simulink library "SimWindFarm_lib"  (Simulink 10.3)
settings: Solver=ode45  StartTime=0.0  StopTime=10.0  RelTol=1e-3  EnableMultiTasking=on
undefined symbols (not defined in the file): sigbuilder_block
libraries: simulink x3
(part 1 of 2)
settings Model: Creator=grunnet  LastModifiedBy=yerai
settings Model: SuppressorTable=|
  | <?xml version="1.0" encoding="UTF-8" standalone="yes" ?>
  | <!DOCTYPE boost_serialization>
  | <boost_serialization signature="serialization::archive" version="17">
  | <DiagnosticSuppressor class_id="0" tracking_level="0" version="7">
  | 	<Table class_id="1" tracking_level="0" version="0">
  | 		<count>3</count>
  | 		<bucket_count>8</bucket_count>
  | 		<item_version>0</item_version>
  | 		<item class_id="2" tracking_level="0" version="0">
  | 			<first class_id="3" tracking_level="0" version="7">
  | 				<Source class_id="4" tracking_level="0" version="0">
  | 					<count>1</count>
  | 					<item_version>0</item_version>
  | 					<item>183</item>
  | 				</Source>
  | 			</first>
  | 			<second class_id="5" tracking_level="0" version="7">
  | 				<SuppressedData class_id="6" tracking_level="0" version="0">
  | 					<count>2</count>
  | 					<bucket_count>8</bucket_count>
  | 					<item_version>0</item_version>
  | 					<item class_id="7" tracking_level="0" version="0">
  | 						<first class_id="8" tracking_level="0" version="7">
  | 							<ID>SimulinkFixedPoint:util:Overflowoccurred</ID>
  | 							<Cause>
  | 								<Source>
  | 									<count>0</count>
  | 									<item_version>0</item_version>
  | 								</Source>
  | 							</Cause>
  | 						</first>
  | 						<second class_id="9" tracking_level="0" version="7">
  | 							<Comment></Comment>
  | 							<User></User>
  | 							<LastModified class_id="10" tracking_level="0" version="0">
  | 								<ptime_date class_id="11" tracking_level="0" version="0">
  | 									<date>20160523</date>
  | 								</ptime_date>
  | 								<ptime_time_duration class_id="12" tracking_level="0" version="1">
  | 									<is_special>0</is_special>
  | 									<time_duration_hours>10</time_duration_hours>
  | 									<time_duration_minutes>57</time_duration_minutes>
  | 									<time_duration_seconds>55</time_duration_seconds>
  | 									<time_duration_fractional_seconds>0</time_duration_fractional_seconds>
  | 								</ptime_time_duration>
  | 							</LastModified>
  | 							<SuppressionType>1</SuppressionType>
  | 						</second>
  | 					</item>
  | 					<item>
  | 						<first>
  | 							<ID>Simulink:DataType:WarningOverFlowDetected</ID>
  | 							<Cause>
  | 								<Source>
  | 									<count>0</count>
  | 									<item_version>0</item_version>
  | 								</Source>
  | 							</Cause>
  | 						</first>
  | 						<second>
  | 							<Comment></Comment>
  | 							<User></User>
  | 							<LastModified>
  | 								<ptime_date>
  | 									<date>20160523</date>
  | 								</ptime_date>
  | 								<ptime_time_duration>
  | 									<is_special>0</is_special>
  | 									<time_duration_hours>10</time_duration_hours>
  | 									<time_duration_minutes>57</time_duration_minutes>
  | 									<time_duration_seconds>55</time_duration_seconds>
  | 									<time_duration_fractional_seconds>0</time_duration_fractional_seconds>
  | 								</ptime_time_duration>
  | 							</LastModified>
  | 							<SuppressionType>1</SuppressionType>
  | 						</second>
  | 					</item>
  | 				</SuppressedData>
  | 			</second>
  | 		</item>
  | 		<item>
  | 			<first>
  | 				<Source>
  | 					<count>1</count>
  | 					<item_version>0</item_version>
  | 					<item>243:183</item>
  | 				</Source>
  | 			</first>
  | 			<second>
  | 				<SuppressedData>
  | 					<count>2</count>
  | 					<bucket_count>8</bucket_count>
  | 					<item_version>0</item_version>
  | 					<item>
  | 						<first>
  | 							<ID>SimulinkFixedPoint:util:Overflowoccurred</ID>
  | 							<Cause>
  | 								<Source>
  | 									<count>0</count>
  | 									<item_version>0</item_version>
  | 								</Source>
  | 							</Cause>
  | 						</first>
  | 						<second>
  | 							<Comment></Comment>
  | 							<User></User>
  | 							<LastModified>
  | 								<ptime_date>
  | 									<date>20160523</date>
  | 								</ptime_date>
  | 								<ptime_time_duration>
  | 									<is_special>0</is_special>
  | 									<time_duration_hours>10</time_duration_hours>
  | 									<time_duration_minutes>57</time_duration_minutes>
  | 									<time_duration_seconds>55</time_duration_seconds>
  | 									<time_duration_fractional_seconds>0</time_duration_fractional_seconds>
  | 								</ptime_time_duration>
  | 							</LastModified>
  | 							<SuppressionType>1</SuppressionType>
  | 						</second>
  | 					</item>
  | 					<item>
  | 						<first>
  | 							<ID>Simulink:DataType:WarningOverFlowDetected</ID>
  | 							<Cause>
  | 								<Source>
  | 									<count>0</count>
  | 									<item_version>0</item_version>
  | 								</Source>
  | 							</Cause>
  | 						</first>
  | 						<second>
  | 							<Comment></Comment>
  | 							<User></User>
  | 							<LastModified>
  | 								<ptime_date>
  | 									<date>20160523</date>
  | 								</ptime_date>
  | 								<ptime_time_duration>
  | 									<is_special>0</is_special>
  | 									<time_duration_hours>10</time_duration_hours>
  | 									<time_duration_minutes>57</time_duration_minutes>
  | 									<time_duration_seconds>55</time_duration_seconds>
  | 									<time_duration_fractional_seconds>0</time_duration_fractional_seconds>
  | 								</ptime_time_duration>
  | 							</LastModified>
  | 							<SuppressionType>1</SuppressionType>
  | 						</second>
  | 					</item>
  | 				</SuppressedData>
  | 			</second>
  | 		</item>
  | 		<item>
  | 			<first>
  | 				<Source>
  | 					<count>1</count>
  | 					<item_version>0</item_version>
  | 					<item>80</item>
  | 				</Source>
  | 			</first>
  | 			<second>
  | 				<SuppressedData>
  | 					<count>2</count>
  | 					<bucket_count>8</bucket_count>
  | 					<item_version>0</item_version>
  | 					<item>
  | 						<first>
  | 							<ID>SimulinkFixedPoint:util:Overflowoccurred</ID>
  | 							<Cause>
  | 								<Source>
  | 									<count>0</count>
  | 									<item_version>0</item_version>
  | 								</Source>
  | 							</Cause>
  | 						</first>
  | 						<second>
  | 							<Comment></Comment>
  | 							<User></User>
  | 							<LastModified>
  | 								<ptime_date>
  | 									<date>20160523</date>
  | 								</ptime_date>
  | 								<ptime_time_duration>
  | 									<is_special>0</is_special>
  | 									<time_duration_hours>10</time_duration_hours>
  | 									<time_duration_minutes>57</time_duration_minutes>
  | 									<time_duration_seconds>55</time_duration_seconds>
  | 									<time_duration_fractional_seconds>0</time_duration_fractional_seconds>
  | 								</ptime_time_duration>
  | 							</LastModified>
  | 							<SuppressionType>1</SuppressionType>
  | 						</second>
  | 					</item>
  | 					<item>
  | 						<first>
  | 							<ID>Simulink:DataType:WarningOverFlowDetected</ID>
  | 							<Cause>
  | 								<Source>
  | 									<count>0</count>
  | 									<item_version>0</item_version>
  | 								</Source>
  | 							</Cause>
  | 						</first>
  | 						<second>
  | 							<Comment></Comment>
  | 							<User></User>
  | 							<LastModified>
  | 								<ptime_date>
  | 									<date>20160523</date>
  | 								</ptime_date>
  | 								<ptime_time_duration>
  | 									<is_special>0</is_special>
  | 									<time_duration_hours>10</time_duration_hours>
  | 									<time_duration_minutes>57</time_duration_minutes>
  | 									<time_duration_seconds>55</time_duration_seconds>
  | 									<time_duration_fractional_seconds>0</time_duration_fractional_seconds>
  | 								</ptime_time_duration>
  | 							</LastModified>
  | 							<SuppressionType>1</SuppressionType>
  | 						</second>
  | 					</item>
  | 				</SuppressedData>
  | 			</second>
  | 		</item>
  | 	</Table>
  | </DiagnosticSuppressor>
  | 
  | </boost_serialization>
  | 
  | </boost_serialization>

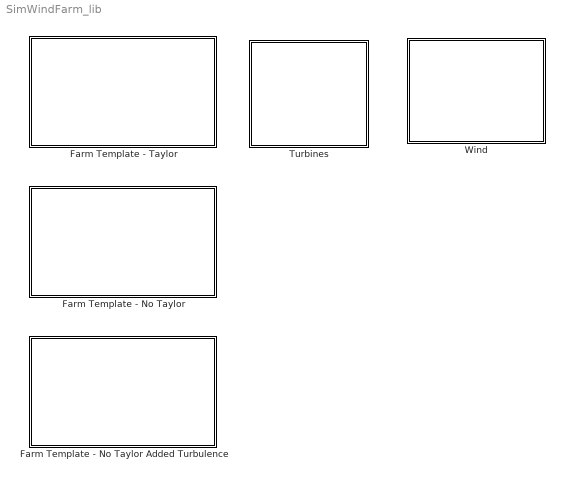
== system SimWindFarm_lib ==
  Farm Template - No Taylor : Subsystem  mask(Aeolus){}
      mask help: Wind Farm Template for the Aeolus Farm Simulator.
      settings: OpenFcn=create_windfarm_no_taylor()
      mask Display: image(imread('farm.jpg'))
  Farm Template - No Taylor Added Turbulence : Subsystem  AncestorBlock=libaeolus_at/Farm Template - No Taylor  mask(Aeolus){}
      mask help: Wind Farm Template for the Aeolus Farm Simulator.
      settings: OpenFcn=create_windfarm_no_taylor()
      mask Display: image(imread('farm.jpg'))
  Farm Template - Taylor : Subsystem  mask(Aeolus){}
      mask help: Wind Farm Template for the Aeolus Farm Simulator.
      settings: OpenFcn=create_windfarm()
      mask Display: image(imread('farm.jpg'))
  Turbines : Subsystem
      settings: OpenFcn=libturbines
      mask Display: image(imread('tblib.jpg'))
  Wind : Subsystem
      settings: OpenFcn=libwind
      mask Display: image(imread('wind.jpg'))

== system SimWindFarm_lib/Farm Template - No Taylor ==
  Farm Control : Subsystem  mask(Farm Control){Ts=5}
      mask prompts: Ts "Control Sample Time"
      mask help: A Farm controller with proportional distribution
      mask init:
      | parm=get_param(gcb,'UserData');
      | CTs=Ts;
      mask Display:
      | color('black')
      | port_label('input',1,'P_meas [W]')
      | port_label('input',2,'V_meas [m/s]')
      | port_label('input',3,'w_rot [rad/s]')
      | port_label('input',4,'Pitch [deg]')
      | port_label('input',5,'Aux')
      | port_label('input',6,'P_farm_dem [W]')
      | 
      | 
      | port_label('output',1,'P_dem[W]')
      | port_label('output',2,'P_avail [W]')
  Grid : Subsystem  mask{fgain=2e-9}
      mask prompts: fgain "Power to frequency gain"
      mask init:
      | frequencygain=fgain;
      mask Display:
      | image(imread('grid.jpg'))
      | 
      | port_label('input',1,'P_farm [W]')
      | port_label('input',2,'P_grid [W]')
      | port_label('output',1,'f_grid [Hz]')
  Network Load : Subsystem  mask{maxp=15e6}
      mask prompts: maxp "Max farm power [W]"
      mask init:
      | maxpower=maxp;
      mask Display:
      | image(imread('load.png'))
      | 
      | port_label('output',1,'P_grid[W]')
  Network Operator : Subsystem  mask{mode=Absolute, Ts=30, pref=12e6, rate=1e6, delta=2e6, db=.1, cb=1, maxp=15e6, minp=10e6, freq=50, delay=.1}
      mask prompts: mode "Operating Mode"; Ts "Sample Time [s]"; pref "Power reference [W]"; rate "Power rate limit [W/s]"; delta "Reserved power [W]"; db "Dead band [Hz]"; cb "Control band [Hz]"; maxp "Maximum power [W]"; minp "Minimum power [W]"; freq "Frequency reference [Hz]"; delay "Communication delay [s]"
      mask help: Network Operator Parameters
      mask init:
      | parm.Ts=Ts;
      | parm.mode=mode;
      | switch(mode)
      |     case 1
      |         parm.settings(1)=pref;
      |     case 2
      |         parm.settings(1)=delta;
      |     case 3
      |         parm.settings(1)=pref;
      |     case 4
      |         parm.settings(1)=rate;
      |     case 5
      |         parm.settings(1)=db;
      |         parm.settings(2)=cb;
      |         parm.settings(3)=maxp;
      |         parm.settings(4)=minp;
      |         parm.settings(5)=freq;
      |     otherwise
      |         parm.settings(1)=1e10;
      | end
      | parm.delay=delay;
      mask TypeOptions mode: Absolute | Delta | Balance | Rate Limit | Frequency
      mask Callback mode:
      | m=get_param(gcb,'mode');
      | switch(m)
      |     case 'Absolute'
      |         mv={'on','on','on','off','off', ...
      |             'off','off','off','off','off','on'};
      |     case 'Delta'
      |         mv={'on','on','off','off','on', ...
      |             'off','off','off','off','off','on'};
      |     case 'Balance'
      |         mv={'on','on','on','off','off', ...
      |             'off','off','off','off','off','on'};
      |     case 'Rate Limit'
      |         mv={'on','on','off','on','off', ...
      |             'off','off','off','off','off','on'};
      |     case 'Frequency'
      |         mv={'on','on','off','off','off', ...
      |             'on','on','on','on','on','on'};
      | end
      | 
      | set_param(gcb,'MaskVisibilities',mv);
      mask Display:
      | port_label('output',1,'P_farm_dem [W]')
      | port_label('input',1,'P_avail[W]')
      | port_label('input',2,'f_grid [Hz]')
  Post processing : Subsystem
      mask Display: image(imread('postproc.png'))
  Total power : Sum  Inputs=+
  Turbines : Subsystem  LoadFcn=|  mask(Data logging setup){mode=Wind Sync, ts=-1, dec=1}
      | p=get_param(gcb,'UserData');                                                                                                                                            
      | %If not compatible                                                                                                                                                      
      |                                                                                                                                                                         
      | %Check to avoid template warning                                                                                                                                        
      | if(~isempty(p))                                                                                                                                                         
      |                                                                                                                                                                         
      | 	if(~iscompat(p.version))                                                                                                                                               
      | 		warndlg('The version of SimWindFarm used to create this model does not match the installed version! This may result in undefined behaviour.','Model version mismatch')
      | 	end                                                                                                                                                                    
      | end
      mask prompts: mode "Sample Mode"; ts "Sample Time"; dec "Decimation"
      mask help: Adjust the amount of data logged from the turbines
      mask init:
      | switch(mode)
      |     case 3 %inherit
      |         TTs=-1;
      |     case 1 %Wind
      |         TTs=str2num(get_param([bdroot '/Wind Field/CTrate'],'OutPortSampleTime'));
      |     case 2 %costum
      |         TTs=ts;
      | end
      | 
      | assignin('base','SWFdecimation',dec);
      | assignin('base','SWFTTs',TTs);
      mask Help:
      | Wind Synch - Data is logged with the wind field time step
      | Specify - Set a custom sampling time
      | Inherit - Inherit from output port
      mask TypeOptions mode: Wind Sync | Specify | Inherit
      mask Callback mode:
      | m=get_param(gcb,'mode');
      | switch(m)
      |     case 'Specify'
      |         mv={'on','on','on'};
      |     otherwise %case 'Wind Sync'
      |         mv={'on','off','on'};
      | end
      | 
      | set_param(gcb,'MaskVisibilities',mv);
      mask Display:
      | image(imread('tblib.jpg'))
      | port_label('input',1,'P_dem [W]')
      | port_label('input',2,'V_rot [m/s]')
      | port_label('input',3,'V_nac [m/s]')
      | port_label('output',1,'P [W]')
      | port_label('output',2,'V_meas [m/s]')
      | port_label('output',3,'w_gen [m/s]')
      | port_label('output',4,'Pitch [deg]')
      | port_label('output',5,'Aux')
      | port_label('output',6,'CT')
  Wind Field : Subsystem
      mask init:
      | p=get_param(gcb,'UserData');
      settings: OpenFcn=|
      | [wfile,wpath,wfidx]=uigetfile('*.mat','Select a Wind Data File');
      | if isequal(wfile,0) || isequal(wpath,0)
      |    return
      | end
      | 
      | %Loads wind profile data
      | l=load([wpath wfile]);
      | p=get_param([gcb '/Ambient Lateral Field'],'UserData');
      | 
      | %Check for compatible wind field
      | if (~isequal(p.grid,l.wind.grid))
      |     str_grids = sprintf('\n            Model     New wind \n size          %d         %d \n xsize       %d       %d \n ysize        %d      %d \n \n Try to type: help create_windfield_no_taylor',p.grid.size, l.wind.grid.size, p.grid.xsize, l.wind.grid.xsize, p.grid.ysize, l.wind.grid.ysize);
      |     errordlg(['The wind fields must have the same grid' str_grids],'Wind field Error')
      |    return
      | end
      | 
      | %Check for correct wind field type
      | if(~isfield(l.wind,'ambient_wind'))
      |     errordlg('It is not the correct wind field type. Probably a normal taylor wind field. See create_windfield_no_taylor()','Wind field invalid')
      |    return
      | end
      | 
      | %Check compatible mean wind speed
      | if(~isfield(l.wind,'Umean') | ~isfield(p,'Umean'))
      |     warning('WarnTests:convertTest','Mean wind speed is not part of wind field struct.\n Consider updating model or windfield to newest version of SimWindFarm \n To get correct simulation behaviour, the mean wind speed of the wind field needs to be equal to the one used when farm model is created')
      | else
      |     if (~isequal(p.Umean,l.wind.Umean))
      |         str_wind_speeds = sprintf('Old mean wind speed (%d m/s) does not correspond to new mean wind speed (%d m/s). \n This may cause the simulation to be incorrect because wake delay between turbines changes. \n The solution is to create a new model with the desired average wind speed. \n Setting new windfield anyway.....', p.Umean, l.wind.Umean);
      |         warndlg(str_wind_speeds, 'Mean wind speed incompatibility')
      |     end
      | end
      | 
      | 
      | 
      | if(~isequal(p.ambient_wind.wind_pos,l.wind.ambient_wind.wind_pos))
      |   errordlg('The turbines must have same position','Wind field Error')
      |    return
      | end
      | 
      | %If the wind field is too short, reset the simulation time
      | if(p.SimTime < eval(get_param(bdroot,'StopTime')))
      |     warndlg('The model simulation time is longer than windfield. Resetting model simulation time')
      |     set_param(bdroot,'StopTime',num2str(p.SimTime))
      | end
      | 
      | 
      | %Change wf sample time
      | set_param([gcb '/CTrate'],'OutPortSampleTime',num2str(l.wind.Ts))
      | 
      | %Add old turbine position data
      | l.wind.xgrids=p.xgrids;
      | 
      | %Save the new parameters
      | set_param([gcb '/Ambient Lateral Field'],'UserData',l.wind);
      | for i=1:length(p.ambient_wind.turb_pos)
      |   pp = get_param([gcb '/Wind Speed'   num2str(i)],'UserData');
      |   pp_new = pp;
      |   pp_new.wind = l.wind.ambient_wind.wind{i};
      |   set_param([gcb '/Wind Speed' num2str(i)],'UserData',pp_new);
      | end
      mask Display:
      | image(imread('wind.jpg'))
      | 
      | port_label('input',1,'CT')
      | port_label('output',1,'V_nac [m/s]')
      | port_label('output',2,'V_rot [m/s]')
  wires:
  Turbines/3(w_gen) -> Farm Control/3(w_rot [rad/s])
  Turbines/4(pitch) -> Farm Control/4(Pitch [deg])
  Turbines/5(aux) -> Farm Control/5(" Aux")
  Network Load/1(Power Consumption [W]) -> Grid/2(Consumed Power [W])
  Total power/1 -> Grid/1(Generated Power [W])
  Grid/1(Grid Frequency [Hz]) -> Network Operator/2(Freq [Hz])
  Network Operator/1(P_farm [W]) -> Farm Control/6(P_farm [W])
  Farm Control/2(P_avail [W]) -> Network Operator/1(P_avail [W])
  Turbines/1(P) -> Farm Control/1(P_meas [W]), Total power/1
  Turbines/2(V_nac_meas [m/s]) -> Farm Control/2(V_meas [m/s])
  Farm Control/1(P_dem [W]) -> Turbines/1(P_dem [W])
  Wind Field/2(V_rot) -> Turbines/2(V_rot [m/s])
  Wind Field/1(V_nac) -> Turbines/3(V_nac [m/s])
  Turbines/6(CT) -> Wind Field/1(CT)

== system SimWindFarm_lib/Farm Template - No Taylor Added Turbulence ==
  Farm Control : Subsystem  mask(Farm Control){Ts=5}
      mask prompts: Ts "Control Sample Time"
      mask help: A Farm controller with proportional distribution
      mask init:
      | parm=get_param(gcb,'UserData');
      | CTs=Ts;
      mask Display:
      | color('black')
      | port_label('input',1,'P_meas [W]')
      | port_label('input',2,'V_meas [m/s]')
      | port_label('input',3,'w_rot [rad/s]')
      | port_label('input',4,'Pitch [deg]')
      | port_label('input',5,'Aux')
      | port_label('input',6,'P_farm_dem [W]')
      | 
      | 
      | port_label('output',1,'P_dem[W]')
      | port_label('output',2,'P_avail [W]')
  Grid : Subsystem  mask{fgain=2e-9}
      mask prompts: fgain "Power to frequency gain"
      mask init:
      | frequencygain=fgain;
      mask Display:
      | image(imread('grid.jpg'))
      | 
      | port_label('input',1,'P_farm [W]')
      | port_label('input',2,'P_grid [W]')
      | port_label('output',1,'f_grid [Hz]')
  Network Load : Subsystem  mask{maxp=15e6}
      mask prompts: maxp "Max farm power [W]"
      mask init:
      | maxpower=maxp;
      mask Display:
      | image(imread('load.png'))
      | 
      | port_label('output',1,'P_grid[W]')
  Network Operator : Subsystem  mask{mode=Absolute, Ts=30, pref=12e6, rate=1e6, delta=2e6, db=.1, cb=1, maxp=15e6, minp=10e6, freq=50, delay=.1}
      mask prompts: mode "Operating Mode"; Ts "Sample Time [s]"; pref "Power reference [W]"; rate "Power rate limit [W/s]"; delta "Reserved power [W]"; db "Dead band [Hz]"; cb "Control band [Hz]"; maxp "Maximum power [W]"; minp "Minimum power [W]"; freq "Frequency reference [Hz]"; delay "Communication delay [s]"
      mask help: Network Operator Parameters
      mask init: same as SimWindFarm_lib/Farm Template - No Taylor/Network Operator
      mask TypeOptions mode: Absolute | Delta | Balance | Rate Limit | Frequency
      mask Callback mode:
      | m=get_param(gcb,'mode');
      | switch(m)
      |     case 'Absolute'
      |         mv={'on','on','on','off','off', ...
      |             'off','off','off','off','off','on'};
      |     case 'Delta'
      |         mv={'on','on','off','off','on', ...
      |             'off','off','off','off','off','on'};
      |     case 'Balance'
      |         mv={'on','on','on','off','off', ...
      |             'off','off','off','off','off','on'};
      |     case 'Rate Limit'
      |         mv={'on','on','off','on','off', ...
      |             'off','off','off','off','off','on'};
      |     case 'Frequency'
      |         mv={'on','on','off','off','off', ...
      |             'on','on','on','on','on','on'};
      | end
      | 
      | set_param(gcb,'MaskVisibilities',mv);
      mask Display:
      | port_label('output',1,'P_farm_dem [W]')
      | port_label('input',1,'P_avail[W]')
      | port_label('input',2,'f_grid [Hz]')
  Post processing : Subsystem
      mask Display: image(imread('postproc.png'))
  Total power : Sum  Inputs=+
  Turbines : Subsystem  LoadFcn=|  mask(Data logging setup){mode=Wind Sync, ts=-1, dec=1}
      | p=get_param(gcb,'UserData');                                                                                                                                            
      | %If not compatible                                                                                                                                                      
      |                                                                                                                                                                         
      | %Check to avoid template warning                                                                                                                                        
      | if(~isempty(p))                                                                                                                                                         
      |                                                                                                                                                                         
      | 	if(~iscompat(p.version))                                                                                                                                               
      | 		warndlg('The version of SimWindFarm used to create this model does not match the installed version! This may result in undefined behaviour.','Model version mismatch')
      | 	end                                                                                                                                                                    
      | end
      mask prompts: mode "Sample Mode"; ts "Sample Time"; dec "Decimation"
      mask help: Adjust the amount of data logged from the turbines
      mask init: same as SimWindFarm_lib/Farm Template - No Taylor/Turbines
      mask Help:
      | Wind Synch - Data is logged with the wind field time step
      | Specify - Set a custom sampling time
      | Inherit - Inherit from output port
      mask TypeOptions mode: Wind Sync | Specify | Inherit
      mask Callback mode:
      | m=get_param(gcb,'mode');
      | switch(m)
      |     case 'Specify'
      |         mv={'on','on','on'};
      |     otherwise %case 'Wind Sync'
      |         mv={'on','off','on'};
      | end
      | 
      | set_param(gcb,'MaskVisibilities',mv);
      mask Display:
      | image(imread('tblib.jpg'))
      | port_label('input',1,'P_dem [W]')
      | port_label('input',2,'V_rot [m/s]')
      | port_label('input',3,'V_nac [m/s]')
      | port_label('output',1,'P [W]')
      | port_label('output',2,'V_meas [m/s]')
      | port_label('output',3,'w_gen [m/s]')
      | port_label('output',4,'Pitch [deg]')
      | port_label('output',5,'Aux')
      | port_label('output',6,'CT')
  Wind Field : Subsystem
      mask init:
      | p=get_param(gcb,'UserData');
      settings: OpenFcn=|
      | [wfile,wpath,wfidx]=uigetfile('*.mat','Select a Wind Data File');
      | if isequal(wfile,0) || isequal(wpath,0)
      |    return
      | end
      | 
      | %Loads wind profile data
      | l=load([wpath wfile]);
      | p=get_param([gcb '/Ambient Lateral Field'],'UserData');
      | 
      | %Check for compatible wind field
      | if (~isequal(p.grid,l.wind.grid))
      |     str_grids = sprintf('\n            Model     New wind \n size          %d         %d \n xsize       %d       %d \n ysize        %d      %d \n \n Try to type: help create_windfield_no_taylor',p.grid.size, l.wind.grid.size, p.grid.xsize, l.wind.grid.xsize, p.grid.ysize, l.wind.grid.ysize);
      |     errordlg(['The wind fields must have the same grid' str_grids],'Wind field Error')
      |    return
      | end
      | 
      | %Check for correct wind field type
      | if(~isfield(l.wind,'ambient_wind'))
      |     errordlg('It is not the correct wind field type. Probably a normal taylor wind field. See create_windfield_no_taylor()','Wind field invalid')
      |    return
      | end
      | 
      | %Check compatible mean wind speed
      | if(~isfield(l.wind,'Umean') | ~isfield(p,'Umean'))
      |     warning('WarnTests:convertTest','Mean wind speed is not part of wind field struct.\n Consider updating model or windfield to newest version of SimWindFarm \n To get correct simulation behaviour, the mean wind speed of the wind field needs to be equal to the one used when farm model is created')
      | else
      |     if (~isequal(p.Umean,l.wind.Umean))
      |         str_wind_speeds = sprintf('Old mean wind speed (%d m/s) does not correspond to new mean wind speed (%d m/s). \n This may cause the simulation to be incorrect because wake delay between turbines changes. \n The solution is to create a new model with the desired average wind speed. \n Setting new windfield anyway.....', p.Umean, l.wind.Umean);
      |         warndlg(str_wind_speeds, 'Mean wind speed incompatibility')
      |     end
      | end
      | 
      | 
      | 
      | if(~isequal(p.ambient_wind.wind_pos,l.wind.ambient_wind.wind_pos))
      |   errordlg('The turbines must have same position','Wind field Error')
      |    return
      | end
      | 
      | %If the wind field is too short, reset the simulation time
      | if(p.SimTime < eval(get_param(bdroot,'StopTime')))
      |     warndlg('The model simulation time is longer than windfield. Resetting model simulation time')
      |     set_param(bdroot,'StopTime',num2str(p.SimTime))
      | end
      | 
      | 
      | %Change wf sample time
      | set_param([gcb '/CTrate'],'OutPortSampleTime',num2str(l.wind.Ts))
      | 
      | %Add old turbine position data
      | l.wind.xgrids=p.xgrids;
      | 
      | %Save the new parameters
      | set_param([gcb '/Ambient Lateral Field'],'UserData',l.wind);
      | for i=1:length(p.ambient_wind.turb_pos)
      |   pp = get_param([gcb '/Wind Speed'   num2str(i)],'UserData');
      |   pp_new = pp;
      |   pp_new.wind = l.wind.ambient_wind.wind{i};
      |   set_param([gcb '/Wind Speed' num2str(i)],'UserData',pp_new);
      | end
      mask Display:
      | image(imread('wind.jpg'))
      | 
      | port_label('input',1,'CT')
      | port_label('output',1,'V_nac [m/s]')
      | port_label('output',2,'V_rot [m/s]')
  wires:
  Turbines/6(CT) -> Wind Field/1(CT)
  Wind Field/1(V_nac) -> Turbines/3(V_nac [m/s])
  Wind Field/2(V_rot) -> Turbines/2(V_rot [m/s])
  Farm Control/1(P_dem [W]) -> Turbines/1(P_dem [W])
  Turbines/2(V_nac_meas [m/s]) -> Farm Control/2(V_meas [m/s])
  Turbines/1(P) -> Total power/1, Farm Control/1(P_meas [W])
  Farm Control/2(P_avail [W]) -> Network Operator/1(P_avail [W])
  Network Operator/1(P_farm [W]) -> Farm Control/6(P_farm [W])
  Grid/1(Grid Frequency [Hz]) -> Network Operator/2(Freq [Hz])
  Total power/1 -> Grid/1(Generated Power [W])
  Network Load/1(Power Consumption [W]) -> Grid/2(Consumed Power [W])
  Turbines/5(aux) -> Farm Control/5(" Aux")
  Turbines/4(pitch) -> Farm Control/4(Pitch [deg])
  Turbines/3(w_gen) -> Farm Control/3(w_rot [rad/s])

== system SimWindFarm_lib/Farm Template - Taylor ==
  Farm Control : Subsystem  mask(Farm Control){Ts=5}
      mask prompts: Ts "Control Sample Time"
      mask help: A Farm controller with proportional distribution
      mask init:
      | parm=get_param(gcb,'UserData');
      | CTs=Ts;
      mask Display:
      | color('black')
      | port_label('input',1,'P_meas [W]')
      | port_label('input',2,'V_meas [m/s]')
      | port_label('input',3,'w_rot [rad/s]')
      | port_label('input',4,'Pitch [deg]')
      | port_label('input',5,'Aux')
      | port_label('input',6,'P_farm_dem [W]')
      | 
      | 
      | port_label('output',1,'P_dem[W]')
      | port_label('output',2,'P_avail [W]')
  Grid : Subsystem  mask{fgain=2e-9}
      mask prompts: fgain "Power to frequency gain"
      mask init:
      | frequencygain=fgain;
      mask Display:
      | image(imread('grid.jpg'))
      | 
      | port_label('input',1,'P_farm [W]')
      | port_label('input',2,'P_grid [W]')
      | port_label('output',1,'f_grid [Hz]')
  Network Load : Subsystem  mask{maxp=15e6}
      mask prompts: maxp "Max farm power [W]"
      mask init:
      | maxpower=maxp;
      mask Display:
      | image(imread('load.png'))
      | 
      | port_label('output',1,'P_grid[W]')
  Network Operator : Subsystem  mask{mode=Absolute, Ts=30, pref=12e6, rate=1e6, delta=2e6, db=.1, cb=1, maxp=15e6, minp=10e6, freq=50, delay=.1}
      mask prompts: mode "Operating Mode"; Ts "Sample Time [s]"; pref "Power reference [W]"; rate "Power rate limit [W/s]"; delta "Reserved power [W]"; db "Dead band [Hz]"; cb "Control band [Hz]"; maxp "Maximum power [W]"; minp "Minimum power [W]"; freq "Frequency reference [Hz]"; delay "Communication delay [s]"
      mask help: Network Operator Parameters
      mask init: same as SimWindFarm_lib/Farm Template - No Taylor/Network Operator
      mask TypeOptions mode: Absolute | Delta | Balance | Rate Limit | Frequency
      mask Callback mode:
      | m=get_param(gcb,'mode');
      | switch(m)
      |     case 'Absolute'
      |         mv={'on','on','on','off','off', ...
      |             'off','off','off','off','off','on'};
      |     case 'Delta'
      |         mv={'on','on','off','off','on', ...
      |             'off','off','off','off','off','on'};
      |     case 'Balance'
      |         mv={'on','on','on','off','off', ...
      |             'off','off','off','off','off','on'};
      |     case 'Rate Limit'
      |         mv={'on','on','off','on','off', ...
      |             'off','off','off','off','off','on'};
      |     case 'Frequency'
      |         mv={'on','on','off','off','off', ...
      |             'on','on','on','on','on','on'};
      | end
      | 
      | set_param(gcb,'MaskVisibilities',mv);
      mask Display:
      | port_label('output',1,'P_farm_dem [W]')
      | port_label('input',1,'P_avail[W]')
      | port_label('input',2,'f_grid [Hz]')
  Post processing : Subsystem
      mask Display: image(imread('postproc.png'))
  Total power : Sum  Inputs=+
  Turbines : Subsystem  LoadFcn=|  mask(Data logging setup){mode=Wind Sync, ts=-1, dec=1}
      | p=get_param(gcb,'UserData');                                                                                                                                            
      | %If not compatible                                                                                                                                                      
      |                                                                                                                                                                         
      | %Check to avoid template warning                                                                                                                                        
      | if(~isempty(p))                                                                                                                                                         
      |                                                                                                                                                                         
      | 	if(~iscompat(p.version))                                                                                                                                               
      | 		warndlg('The version of SimWindFarm used to create this model does not match the installed version! This may result in undefined behaviour.','Model version mismatch')
      | 	end                                                                                                                                                                    
      | end
      mask prompts: mode "Sample Mode"; ts "Sample Time"; dec "Decimation"
      mask help: Adjust the amount of data logged from the turbines
      mask init: same as SimWindFarm_lib/Farm Template - No Taylor/Turbines
      mask Help:
      | Wind Synch - Data is logged with the wind field time step
      | Specify - Set a custom sampling time
      | Inherit - Inherit from output port
      mask TypeOptions mode: Wind Sync | Specify | Inherit
      mask Callback mode:
      | m=get_param(gcb,'mode');
      | switch(m)
      |     case 'Specify'
      |         mv={'on','on','on'};
      |     otherwise %case 'Wind Sync'
      |         mv={'on','off','on'};
      | end
      | 
      | set_param(gcb,'MaskVisibilities',mv);
      mask Display:
      | image(imread('tblib.jpg'))
      | port_label('input',1,'P_dem [W]')
      | port_label('input',2,'V_rot [m/s]')
      | port_label('input',3,'V_nac [m/s]')
      | port_label('output',1,'P [W]')
      | port_label('output',2,'V_meas [m/s]')
      | port_label('output',3,'w_gen [m/s]')
      | port_label('output',4,'Pitch [deg]')
      | port_label('output',5,'Aux')
      | port_label('output',6,'CT')
  Wind Field : Subsystem
      settings: OpenFcn=|
      | [wfile,wpath,wfidx]=uigetfile('*.mat','Select a Wind Data File');
      | if isequal(wfile,0) || isequal(wpath,0)
      |    return
      | end
      | 
      | %Loads wind profile data
      | l=load([wpath wfile]);
      | p=get_param([gcb '/Ambient Field'],'UserData');
      | 
      | %Check compatible mean wind speed
      | if(~isfield(l.wind,'Umean') | ~isfield(p,'Umean'))
      |     warning('WarnTests:convertTest','Mean wind speed is not part of wind field struct.\n Consider updating model or windfield to newest version of SimWindFarm \n To get correct simulation behaviour, the mean wind speed of the wind field needs to be equal to the one used when farm model is created')
      | else
      |     if (~isequal(p.Umean,l.wind.Umean))
      |         str_wind_speeds = sprintf('Old mean wind speed (%d m/s) does not correspond to new mean wind speed (%d m/s). \n This may cause the simulation to be incorrect because wake delay between turbines changes. \n The solution is to create a new model with the desired average wind speed. \n Setting new windfield anyway.....', p.Umean, l.wind.Umean);
      |         warndlg(str_wind_speeds, 'Mean wind speed incompatibility')
      |     end
      | end
      | 
      | %Check for correct wind field type
      | if(isfield(l.wind,'ambient_wind'))
      |     errordlg('It is not the correct wind field type. Probably a no_taylor type wind field. See create_windfield()','Wind field invalid')
      |    return
      | end
      | 
      | %Check for compatible wind field
      | if (~isequal(p.grid,l.wind.grid))
      |     str_grids = sprintf('\n            Model     New wind \n size          %d         %d \n xsize       %d       %d \n ysize        %d      %d \n Try to type: help create_windfield',p.grid.size, l.wind.grid.size, p.grid.xsize, l.wind.grid.xsize, p.grid.ysize, l.wind.grid.ysize);
      |     errordlg(['The wind fields must have the same grid' str_grids],'Wind field Error')
      |    return
      | end
      | 
      | %If the wind field is too short, reset the simulation time
      | if(p.SimTime < eval(get_param(bdroot,'StopTime')))
      |     warndlg('The model simulation time is longer than windfield. Resetting model simulation time')
      |     set_param(bdroot,'StopTime',num2str(p.SimTime))
      | end
      | 
      | %Change wf sample time
      | set_param([gcb '/CTrate'],'OutPortSampleTime',num2str(l.wind.Ts))
      | 
      | %Add old turbine position data
      | l.wind.xgrids=p.xgrids;
      | 
      | %Save the new parameters
      | set_param([gcb '/Ambient Field'],'UserData',l.wind);
      mask Display:
      | image(imread('wind.jpg'))
      | 
      | port_label('input',1,'CT')
      | port_label('output',1,'V_nac [m/s]')
      | port_label('output',2,'V_rot [m/s]')
  wires:
  Turbines/6(CT) -> Wind Field/1(CT)
  Wind Field/1(V_nac [m/s]) -> Turbines/3(V_nac [m/s])
  Wind Field/2(V_rot [m/s]) -> Turbines/2(V_rot [m/s])
  Farm Control/1(P_dem [W]) -> Turbines/1(P_dem [W])
  Turbines/2(V_nac_meas [m/s]) -> Farm Control/2(V_meas [m/s])
  Turbines/1(P) -> Total power/1, Farm Control/1(P_meas [W])
  Farm Control/2(P_avail [W]) -> Network Operator/1(P_avail [W])
  Network Operator/1(P_farm [W]) -> Farm Control/6(P_farm [W])
  Grid/1(Grid Frequency [Hz]) -> Network Operator/2(Freq [Hz])
  Total power/1 -> Grid/1(Generated Power [W])
  Network Load/1(Power Consumption [W]) -> Grid/2(Consumed Power [W])
  Turbines/5(aux) -> Farm Control/5(" Aux")
  Turbines/4(pitch) -> Farm Control/4(Pitch [deg])
  Turbines/3(w_gen) -> Farm Control/3(w_rot [rad/s])

== system SimWindFarm_lib/Turbines ==

== system SimWindFarm_lib/Wind ==

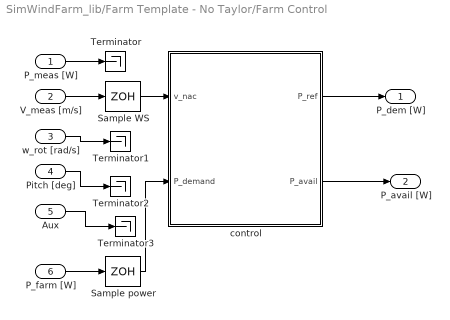
== system SimWindFarm_lib/Farm Template - No Taylor/Farm Control ==
  P_meas [W] : Inport
  V_meas [m/s] : Inport  Port=2
  w_rot [rad/s] : Inport  Port=3
  Pitch [deg] : Inport  Port=4
  " Aux" : Inport  Port=5
  P_farm [W] : Inport  Port=6
  Sample WS : ZeroOrderHold  SampleTime=CTs
  Sample power : ZeroOrderHold  SampleTime=CTs
  Terminator{,1..3} (4 alike) : Terminator
  control : MATLAB Function  TreatAsAtomicUnit=on
  P_dem [W] : Outport
  P_avail [W] : Outport  Port=2
  wires:
  " Aux"/1 -> Terminator3/1
  Pitch [deg]/1 -> Terminator2/1
  w_rot [rad/s]/1 -> Terminator1/1
  P_meas [W]/1 -> Terminator/1
  Sample WS/1 -> control/1(v_nac)
  V_meas [m/s]/1 -> Sample WS/1
  Sample power/1 -> control/2(P_demand)
  control/2(P_avail) -> P_avail [W]/1
  control/1(P_ref) -> P_dem [W]/1
  P_farm [W]/1 -> Sample power/1

== system SimWindFarm_lib/Farm Template - No Taylor/Grid ==
  Generated Power [W] : Inport
  Consumed Power [W] : Inport  Port=2
  Active power diff to freq : Gain  Gain=frequencygain
  Integrator : Integrator  InitialCondition=50  LimitOutput=on  UpperSaturationLimit=100  LowerSaturationLimit=0
  Sum1 : Sum  Inputs=|+-
  Grid Frequency [Hz] : Outport
  wires:
  Consumed Power [W]/1 -> Sum1/2
  Generated Power [W]/1 -> Sum1/1
  Active power diff to freq/1 -> Integrator/1
  Sum1/1 -> Active power diff to freq/1
  Integrator/1 -> Grid Frequency [Hz]/1

== system SimWindFarm_lib/Farm Template - No Taylor/Network Load ==
  Power Load : Subsystem  Tag=STV Subsys  LoadFcn=sigbuilder_block('load');  StartFcn=sigbuilder_block('start');  StopFcn=sigbuilder_block('stop');  ClipboardFcn=sigbuilder_block('clipboard');  mask(Sigbuilder block){tuvar=[0:10]}
      mask help: Sigbuilder GUI
      mask init:
      | if ~strcmp(get_param(bdroot(gcbh),'SimulationStatus'),'stopped') tuvar = sigbuilder_block('maskInit'); end
      settings: CopyFcn=sigbuilder_block('copy');  DeleteFcn=sigbuilder_block('delete');  ModelCloseFcn=sigbuilder_block('modelClose');  PreSaveFcn=sigbuilder_block('preSave');  PauseFcn=sigbuilder_block('pause')  ContinueFcn=sigbuilder_block('continue')  NameChangeFcn=sigbuilder_block('namechange');  OpenFcn=sigbuilder_block('open',[437.6 199.2 550.4 400 ]);  CloseFcn=sigbuilder_block('close');
      mask Display: plot(0, 0, 100, 100,[2, 2, 32, 32, 2], [68, 8, 8, 68, 68],[32, 2], [38, 38], [32, 19, 2],[53, 60, 44], [32, 17, 17, 2],[16, 16, 31, 31]);txt = getActiveGroup(gcbh);text(2, 100, txt,'verticalAlignment', 'top');
  To rated farm power : Gain  Gain=maxpower
  Power Consumption [W] : Outport
  wires:
  To rated farm power/1 -> Power Consumption [W]/1
  Power Load/1(Signal 1) -> To rated farm power/1

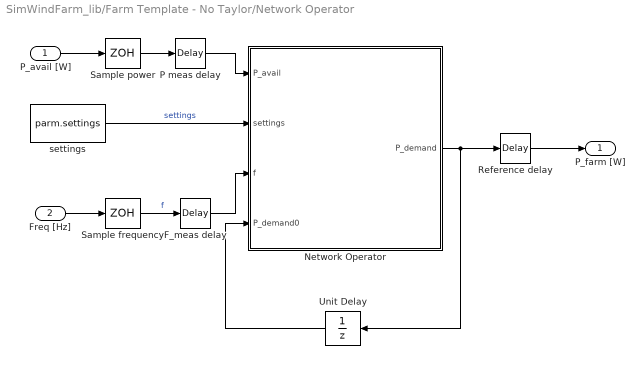
== system SimWindFarm_lib/Farm Template - No Taylor/Network Operator ==
  P_avail [W] : Inport
  Freq [Hz] : Inport  Port=2
  F_meas delay : TransportDelay  DelayTime=parm.delay
  Network Operator : MATLAB Function  TreatAsAtomicUnit=on
  P meas delay : TransportDelay  DelayTime=parm.delay
  Reference delay : TransportDelay  DelayTime=.01
  Sample frequency : ZeroOrderHold  SampleTime=parm.Ts
  Sample power : ZeroOrderHold  SampleTime=parm.Ts
  Unit Delay : UnitDelay  SampleTime=parm.Ts  HasFrameUpgradeWarning=on
  settings : Constant  Value=parm.settings  OutDataTypeStr=double  SampleTime=parm.Ts
  P_farm [W] : Outport
  wires:
  Reference delay/1 -> P_farm [W]/1
  P meas delay/1 -> Network Operator/1(P_avail)
  F_meas delay/1 -> Network Operator/3(f)
  Network Operator/1(P_demand) -> Reference delay/1, Unit Delay/1
  P_avail [W]/1 -> Sample power/1
  Sample power/1 -> P meas delay/1
  settings/1 -> Network Operator/2(settings)  "settings"
  Sample frequency/1 -> F_meas delay/1  "f"
  Unit Delay/1 -> Network Operator/4(P_demand0)
  Freq [Hz]/1 -> Sample frequency/1

== system SimWindFarm_lib/Farm Template - No Taylor/Post processing ==
  Fatigue Computation : Subsystem
      settings: OpenFcn=fatigue=fatiguegui(logsout);
      mask Display: image(imread('rainflow.png'))

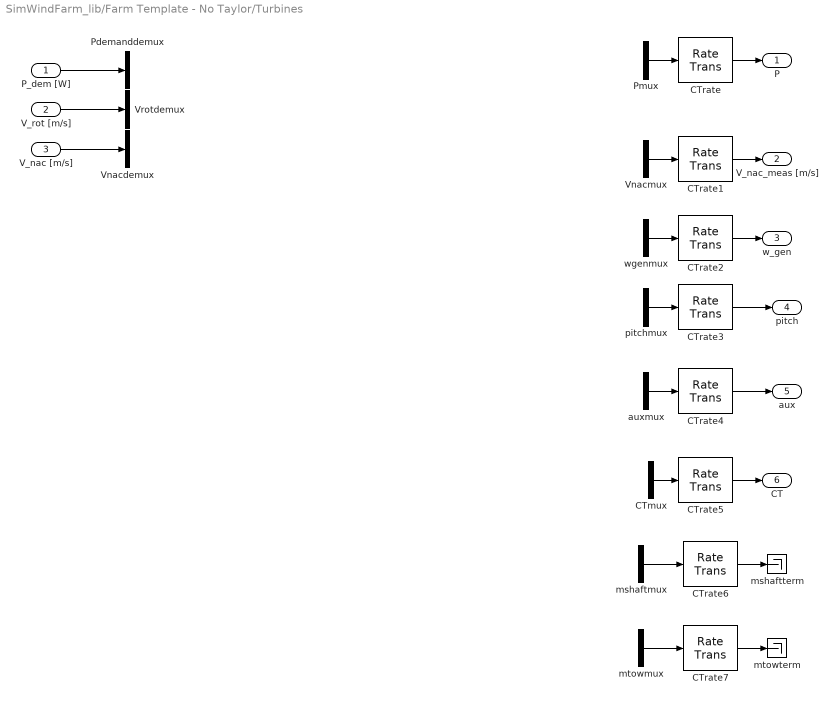
== system SimWindFarm_lib/Farm Template - No Taylor/Turbines ==
  P_dem [W] : Inport
  V_rot [m/s] : Inport  Port=2
  V_nac [m/s] : Inport  Port=3
  CTmux : Mux  Inputs=2
  CTrate{,1..7} (8 alike) : RateTransition  Deterministic=off  OutPortSampleTime=TTs
  Pdemanddemux : Demux  Outputs=3
  Pmux : Mux  Inputs=2
  Vnacdemux : Demux  Outputs=3
  Vnacmux : Mux  Inputs=2
  Vrotdemux : Demux  Outputs=3
  auxmux : Mux  Inputs=2
  mshaftmux : Mux  Inputs=2
  mshaftterm : Terminator
  mtowmux : Mux  Inputs=2
  mtowterm : Terminator
  pitchmux : Mux  Inputs=2
  wgenmux : Mux  Inputs=2
  P : Outport
  V_nac_meas [m/s] : Outport  Port=2
  w_gen : Outport  Port=3
  pitch : Outport  Port=4
  aux : Outport  Port=5
  CT : Outport  Port=6
  wires:
  CTrate7/1 -> mtowterm/1
  CTrate6/1 -> mshaftterm/1
  CTrate5/1 -> CT/1
  CTrate4/1 -> aux/1
  CTrate3/1 -> pitch/1
  CTrate2/1 -> w_gen/1
  CTrate1/1 -> V_nac_meas [m/s]/1
  CTrate/1 -> P/1
  mtowmux/1 -> CTrate7/1
  mshaftmux/1 -> CTrate6/1
  wgenmux/1 -> CTrate2/1
  auxmux/1 -> CTrate4/1
  pitchmux/1 -> CTrate3/1
  Vnacmux/1 -> CTrate1/1
  CTmux/1 -> CTrate5/1
  Pmux/1 -> CTrate/1
  V_rot [m/s]/1 -> Vrotdemux/1
  P_dem [W]/1 -> Pdemanddemux/1
  V_nac [m/s]/1 -> Vnacdemux/1

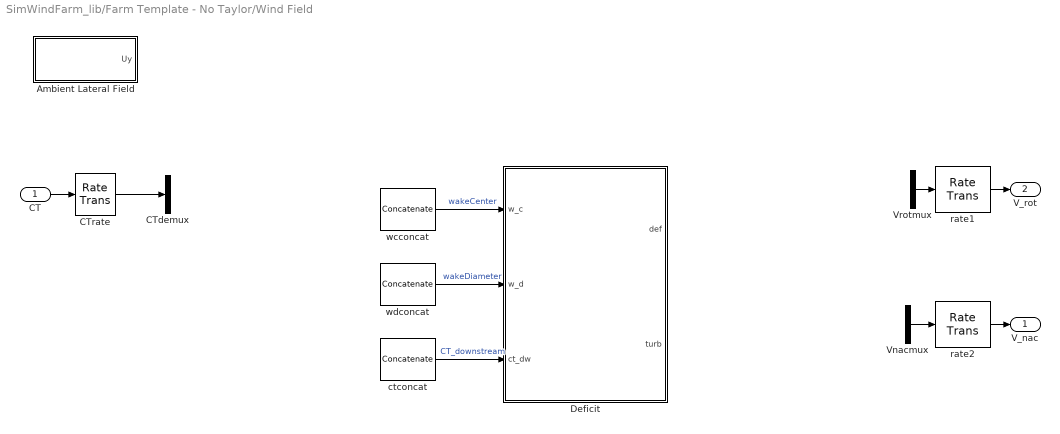
== system SimWindFarm_lib/Farm Template - No Taylor/Wind Field ==
  CT : Inport
  Ambient Lateral Field : Subsystem
      mask init:
      | wind=get_param(gcb,'UserData');
  CTdemux : Demux  Outputs=3
  CTrate : RateTransition  Deterministic=off  OutPortSampleTime=10
  Deficit : MATLAB Function  TreatAsAtomicUnit=on
  Vnacmux : Mux  Inputs=2
  Vrotmux : Mux  Inputs=2
  ctconcat : Concatenate  Mode=Multidimensional array  ConcatenateDimension=2
  rate1 : RateTransition  Deterministic=off  OutPortSampleTime=SWFTTs
  rate2 : RateTransition  Deterministic=off  OutPortSampleTime=SWFTTs
  wcconcat : Concatenate  Mode=Multidimensional array  ConcatenateDimension=2
  wdconcat : Concatenate  Mode=Multidimensional array  ConcatenateDimension=2
  V_nac : Outport
  V_rot : Outport  Port=2
  wires:
  CTrate/1 -> CTdemux/1
  CT/1 -> CTrate/1
  wcconcat/1 -> Deficit/1(w_c)  "wakeCenter"
  wdconcat/1 -> Deficit/2(w_d)  "wakeDiameter"
  ctconcat/1 -> Deficit/3(ct_dw)  "CT_downstream"
  Vrotmux/1 -> rate1/1
  Vnacmux/1 -> rate2/1
  rate1/1 -> V_rot/1
  rate2/1 -> V_nac/1

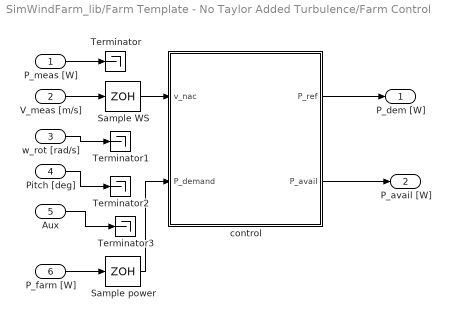
== system SimWindFarm_lib/Farm Template - No Taylor Added Turbulence/Farm Control ==
  P_meas [W] : Inport
  V_meas [m/s] : Inport  Port=2
  w_rot [rad/s] : Inport  Port=3
  Pitch [deg] : Inport  Port=4
  " Aux" : Inport  Port=5
  P_farm [W] : Inport  Port=6
  Sample WS : ZeroOrderHold  SampleTime=CTs
  Sample power : ZeroOrderHold  SampleTime=CTs
  Terminator{,1..3} (4 alike) : Terminator
  control : MATLAB Function  TreatAsAtomicUnit=on
  P_dem [W] : Outport
  P_avail [W] : Outport  Port=2
  wires:
  P_farm [W]/1 -> Sample power/1
  control/1(P_ref) -> P_dem [W]/1
  control/2(P_avail) -> P_avail [W]/1
  Sample power/1 -> control/2(P_demand)
  V_meas [m/s]/1 -> Sample WS/1
  Sample WS/1 -> control/1(v_nac)
  P_meas [W]/1 -> Terminator/1
  w_rot [rad/s]/1 -> Terminator1/1
  Pitch [deg]/1 -> Terminator2/1
  " Aux"/1 -> Terminator3/1

== system SimWindFarm_lib/Farm Template - No Taylor Added Turbulence/Grid ==
  Generated Power [W] : Inport
  Consumed Power [W] : Inport  Port=2
  Active power diff to freq : Gain  Gain=frequencygain
  Integrator : Integrator  InitialCondition=50  LimitOutput=on  UpperSaturationLimit=100  LowerSaturationLimit=0
  Sum1 : Sum  Inputs=|+-
  Grid Frequency [Hz] : Outport
  wires:
  Integrator/1 -> Grid Frequency [Hz]/1
  Sum1/1 -> Active power diff to freq/1
  Active power diff to freq/1 -> Integrator/1
  Generated Power [W]/1 -> Sum1/1
  Consumed Power [W]/1 -> Sum1/2

== system SimWindFarm_lib/Farm Template - No Taylor Added Turbulence/Network Load ==
  Power Load : Subsystem  Tag=STV Subsys  LoadFcn=sigbuilder_block('load');  StartFcn=sigbuilder_block('start');  StopFcn=sigbuilder_block('stop');  ClipboardFcn=sigbuilder_block('clipboard');  mask(Sigbuilder block){tuvar=[0:10]}
      mask help: Sigbuilder GUI
      mask init:
      | if ~strcmp(get_param(bdroot(gcbh),'SimulationStatus'),'stopped') tuvar = sigbuilder_block('maskInit'); end
      settings: CopyFcn=sigbuilder_block('copy');  DeleteFcn=sigbuilder_block('delete');  ModelCloseFcn=sigbuilder_block('modelClose');  PreSaveFcn=sigbuilder_block('preSave');  PauseFcn=sigbuilder_block('pause')  ContinueFcn=sigbuilder_block('continue')  NameChangeFcn=sigbuilder_block('namechange');  OpenFcn=sigbuilder_block('open',[437.6 199.2 550.4 400 ]);  CloseFcn=sigbuilder_block('close');
      mask Display: plot(0, 0, 100, 100,[2, 2, 32, 32, 2], [68, 8, 8, 68, 68],[32, 2], [38, 38], [32, 19, 2],[53, 60, 44], [32, 17, 17, 2],[16, 16, 31, 31]);txt = getActiveGroup(gcbh);text(2, 100, txt,'verticalAlignment', 'top');
  To rated farm power : Gain  Gain=maxpower
  Power Consumption [W] : Outport
  wires:
  Power Load/1(Signal 1) -> To rated farm power/1
  To rated farm power/1 -> Power Consumption [W]/1

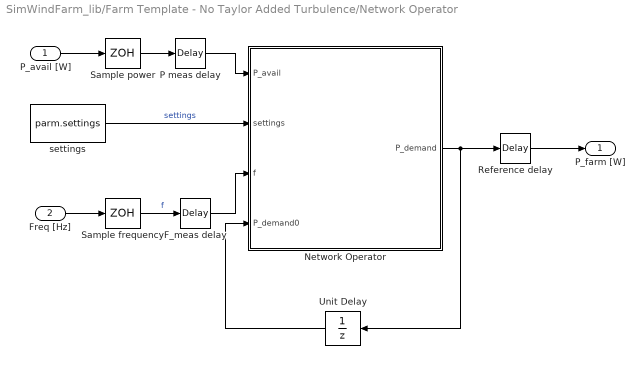
== system SimWindFarm_lib/Farm Template - No Taylor Added Turbulence/Network Operator ==
  P_avail [W] : Inport
  Freq [Hz] : Inport  Port=2
  F_meas delay : TransportDelay  DelayTime=parm.delay
  Network Operator : MATLAB Function  TreatAsAtomicUnit=on
  P meas delay : TransportDelay  DelayTime=parm.delay
  Reference delay : TransportDelay  DelayTime=.01
  Sample frequency : ZeroOrderHold  SampleTime=parm.Ts
  Sample power : ZeroOrderHold  SampleTime=parm.Ts
  Unit Delay : UnitDelay  SampleTime=parm.Ts  HasFrameUpgradeWarning=on
  settings : Constant  Value=parm.settings  OutDataTypeStr=double  SampleTime=parm.Ts
  P_farm [W] : Outport
  wires:
  Freq [Hz]/1 -> Sample frequency/1
  Unit Delay/1 -> Network Operator/4(P_demand0)
  Sample frequency/1 -> F_meas delay/1  "f"
  settings/1 -> Network Operator/2(settings)  "settings"
  Sample power/1 -> P meas delay/1
  P_avail [W]/1 -> Sample power/1
  Network Operator/1(P_demand) -> Unit Delay/1, Reference delay/1
  F_meas delay/1 -> Network Operator/3(f)
  P meas delay/1 -> Network Operator/1(P_avail)
  Reference delay/1 -> P_farm [W]/1
